simulink model "pendulum_animation"  (Simulink 8.2)
settings: Solver=ode45  StartTime=0.0  StopTime=8  RelTol=1e-3
values from neighbouring files (symbols this model uses):
  P = Pinv^(-1)    [controller_pp.m]
undefined symbols (not defined in the file or in its folder): controller, drawPendulum
settings Model: Creator=beard  LastModifiedBy=Priyanka Das
settings OptimizationCC: InitFltsAndDblsToZero=on

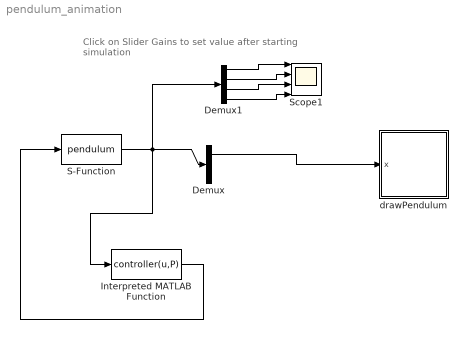
== system pendulum_animation ==
  note: Click on Slider Gains to set value
      | after starting simulation
  Demux : Demux  Outputs=2
  Demux1 : Demux
  Interpreted MATLAB Function : MATLABFcn  MATLABFcn=controller(u,P)
  S-Function : S-Function  FunctionName=pendulum  Parameters=P  EnableBusSupport=off
  Scope1 : Scope  NumInputPorts=4
      settings: TimeRange=200  YMin=-0.178~-1.605~0.01475~0.005  YMax=-0.17~-1.598~0.0175~0.025
  drawPendulum : Subsystem
      mask init:
      | % drawing parameters
      | L = 1;
      | gap = 0.01;
      | width = 1.0;
      | height = 0.1;
      mask Display: image(imread('tv.jpg'))
  wires:
  S-Function/1 -> Demux1/1, Interpreted MATLAB Function/1, Demux/1
  Demux/1 -> drawPendulum/1(x)
  Interpreted MATLAB Function/1 -> S-Function/1
  Demux1/1 -> Scope1/1
  Demux1/2 -> Scope1/2
  Demux1/3 -> Scope1/3
  Demux1/4 -> Scope1/4

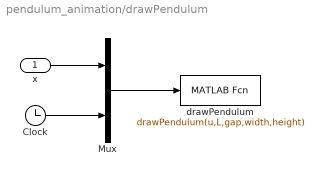
== system pendulum_animation/drawPendulum ==
  x : Inport
  Clock : Clock
  Mux : Mux  Inputs=2
  drawPendulum : MATLABFcn  MATLABFcn=drawPendulum(u,L,gap,width,height)  OutputDimensions=0  SampleTime=0.1
  wires:
  Mux/1 -> drawPendulum/1
  x/1 -> Mux/1
  Clock/1 -> Mux/2
